simulink model "rxTestHarnessSimulinkSide"  (R2021a)
settings: Solver=FixedStepDiscrete  StartTime=0.0  StopTime=10.0  RelTol=1e-3
libraries: hdlsllib x13
settings Model: Creator=cyarp  LastModifiedBy=cyarp

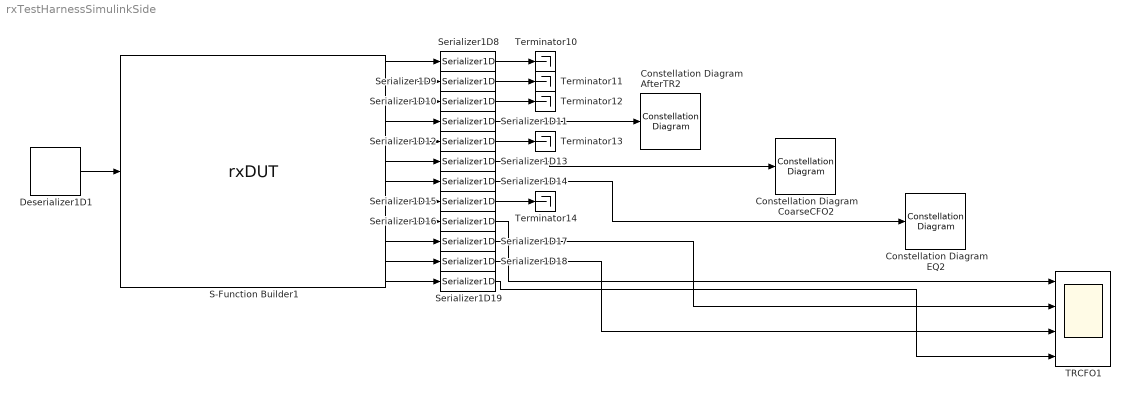
== system rxTestHarnessSimulinkSide ==
  Constellation Diagram AfterTR2 : ConstellationDiagram
  Constellation Diagram CoarseCFO2 : ConstellationDiagram
  Constellation Diagram EQ2 : ConstellationDiagram
  Deserializer1D1 : hdlsllib/HDL Operations/Deserializer1D  Ratio=120  IdleCycles=0  InitialCondition=0  startIn=off  validIn=off  validOut=off  inputDataDimensions=-1  inputSampleTime=-1  inputSignalType=auto
      settings: SourceProductBaseCode=SL
  S-Function Builder1 : S-Function  FunctionName=rxDUT  SFunctionModules=rxDUT_wrapper  SFunctionDeploymentMode=off  EnableBusSupport=off  mask(S-Function Builder){}
      mask help: Simulink:masks:SFunctionBuilder_MD
      mask init:
      | val = [[.9  0.75 0.75 1 1 .9 .9 1]',[1 1 0.75 0.75 .9 .9 1 .9]'];try , sys = get_param(gcb,'SfunBuilderFcnName');if isempty(sys), sys = get_param(gcb,'FunctionName'); end,catch, sys = get_param(gcb,'FunctionName'); end
      settings: CopyFcn=set_param(gcbh,'LinkStatus','none')  OpenFcn=sfunctionwizard(gcbh)
      mask Display: plot(val(:,1),val(:,2)),disp(sys),port_label('input',1,'samplesIn'),port_label('output',1,'dataPacked'),port_label('output',2,'dataPackedValid'),port_label('output',3,'dataPackedLast'),port_label('output',4,'afterTR'),port_label('output',5,'afterTRValid'),port_label('output',6,'coarseCFO'),port_label('output',7,'constPt'),port_label('output',8,'constPtValid'),port_label('output',9,'receiving'),port_label('output',10,'lastPeriod'),port_label('output',11,'trEstDone'),port_label('output',12,'peakCount')
  Serializer1D{8..15} (8 alike) : hdlsllib/HDL Operations/Serializer1D  Ratio=40  IdleCycles=0  validIn=off  startOut=off  validOut=off  inputDataDimensions=-1  inputSampleTime=-1  inputSignalType=auto
      settings: SourceProductBaseCode=SL
  Serializer1D{16..19} (4 alike) : hdlsllib/HDL Operations/Serializer1D  Ratio=120  IdleCycles=0  validIn=off  startOut=off  validOut=off  inputDataDimensions=-1  inputSampleTime=-1  inputSignalType=auto
      settings: SourceProductBaseCode=SL
  TRCFO1 : Scope  NumInputPorts=4
  Terminator{10..14} (5 alike) : Terminator
  wires:
  S-Function Builder1/9 -> Serializer1D16/1
  S-Function Builder1/3 -> Serializer1D10/1
  Serializer1D16/1 -> TRCFO1/1
  Serializer1D18/1 -> TRCFO1/3
  Serializer1D19/1 -> TRCFO1/4
  S-Function Builder1/5 -> Serializer1D12/1
  S-Function Builder1/2 -> Serializer1D9/1
  Serializer1D11/1 -> Constellation Diagram AfterTR2/1
  S-Function Builder1/7 -> Serializer1D14/1
  S-Function Builder1/1 -> Serializer1D8/1
  S-Function Builder1/6 -> Serializer1D13/1
  Serializer1D17/1 -> TRCFO1/2
  Serializer1D14/1 -> Constellation Diagram EQ2/1
  Serializer1D12/1 -> Terminator13/1
  Serializer1D13/1 -> Constellation Diagram CoarseCFO2/1
  S-Function Builder1/8 -> Serializer1D15/1
  Serializer1D10/1 -> Terminator12/1
  S-Function Builder1/10 -> Serializer1D17/1
  S-Function Builder1/12 -> Serializer1D19/1
  S-Function Builder1/11 -> Serializer1D18/1
  ? -> Deserializer1D1/1
  Serializer1D15/1 -> Terminator14/1
  Serializer1D8/1 -> Terminator10/1
  Serializer1D9/1 -> Terminator11/1
  Deserializer1D1/1 -> S-Function Builder1/1
  S-Function Builder1/4 -> Serializer1D11/1
